simulink model "testmodel_gUSBampCSPbci_TwoClass_gOrthosis"  (R2015a)
settings: Solver=FixedStepDiscrete  StartTime=0.0  StopTime=inf  FixedStep=1/256  RelTol=1e-3
InitFcn:
  | global FeedbackGain;
  | FeedbackGain = 0.1;
  | 
  | if exist('WV') ~= 1
  | global WV
  | WV = zeros(1, 5);
  | end
  | 
  | SelectedChannels = str2num(get_param([gcs,'/Select Channels'],'selectedchannels'));
  | NumberOfChannels = length(SelectedChannels);
  | if (exist('W_CSP') ~= 1)
  |     global W_CSP
  |     if NumberOfChannels == 63
  |         try
  |            SPF = spf;
  |            Filter=load(SPF,'generic_CSP_2Class_63channels.mat');
  |            sf = get(Filter,'spf');
  |            spf_struct = struct(sf);
  |            W_CSP = spf_struct.D.W;
  |         catch
  |             W_CSP = zeros(NumberOfChannels,NumberOfChannels);
  |         end
  |     elseif NumberOfChannels == 27
  |         try
  |             W_CSPt = load('template_W_CSP_TwoClasses_27Ch');
  |             W_CSP = W_CSPt.W_CSP;
  |         catch
  |             W_CSP = zeros(NumberOfChannels,NumberOfChannels);
  |         end
  | elseif NumberOfChannels == 16
  |         try
  |             W_CSPt = load('template_W_CSP_TwoClasses_16Ch');
  |             W_CSP = W_CSPt.W_CSP;
  |         catch
  |             W_CSP = zeros(NumberOfChannels,NumberOfChannels);
  |         end
  |     else
  |         W_CSP = zeros(NumberOfChannels,NumberOfChannels);
  |     end
  | end
StartFcn:
  | SelectedChannels = str2num(get_param([gcs,'/Select Channels'],'selectedchannels'));
  | NumberOfChannels = length(SelectedChannels);
  | 
  | NumCsps = size(W_CSP,1);
  | 
  | if (NumCsps ~= NumberOfChannels)
  | troubles('The number of selected channels does not fit to the number of channels used for setting up the CSPs',['Select the channels in the Select Channels -block to get ',num2str(NumCsps),' channels. If you have changed the electrode configuration please restart Matlab.']);
  | set_param(gcs, 'SimulationCommand', 'stop');
  | end
undefined symbols (not defined in the file or in its folder): Filtera, Filterb
libraries: gRTanalyze x5, gtecHighspeedLib x5, recoveriXExtension_Lib x2, OrthosisLib x1
Description:
  | g.USBamp based CSP MI BCI for two classes
  | 
  | Copyright g.tec medical engineering GmbH
settings Model: ModifiedByFormat=g.tec  CovSFcnEnable=off  Creator=g.tec medical engineering GmbH  LastModifiedBy=g.tec
settings DataIOCC: SignalLoggingSaveFormat=ModelDataLogs
settings OptimizationCC: BlockReduction=off  ExpressionDepthLimit=2147483647  InitFltsAndDblsToZero=on
settings DebuggingCC: SaveWithParameterizedLinksMsg=none  UnderspecifiedInitializationDetection=Classic  MergeDetectMultiDrivingBlocksExec=none  SolverPrmCheckMsg=warning  FcnCallInpInsideContextMsg=UseLocalSettings  StateNameClashWarn=warning
settings GRTTargetCC: CombineOutputUpdateFcns=off  GRTInterface=on

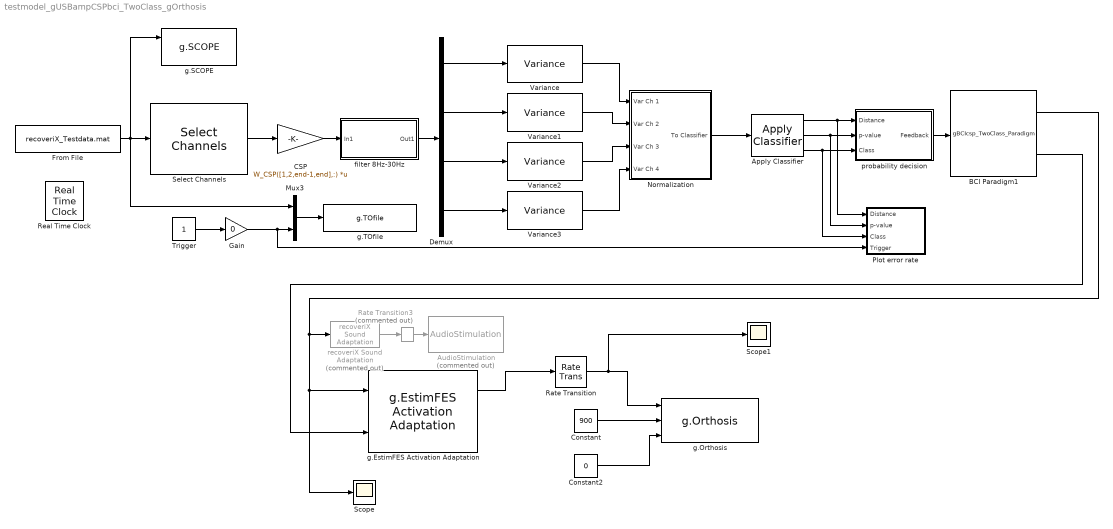
== system testmodel_gUSBampCSPbci_TwoClass_gOrthosis ==
  Apply Classifier : gRTanalyze/Apply Classifier
  AudioStimulation : gtecHighspeedLib/AudioStimulation  Commented=on  audiofiles={'C:\Program Files\gtec\recoveriX g.EstimFES\AudioFiles\Italian\left_resampled.wav' 'C:\Program Files\gtec\recoveriX g.EstimFES\AudioFiles\Italian\right_resampled.wav' 'C:\Program Files\gtec\recoveriX g.EstimFES\AudioFiles\Italian\relax_resampled.wav'}  onsettrigger=0
  BCI Paradigm1 : M-S-Function  FunctionName=gBCIcsp_TwoClass_Paradigm  Parameters=paradigm, runnumber  mask(BCI Paradigm Block){paradigm=feedback, runnumber=1}
      mask TypeOptions paradigm: no feedback | feedback | ball
      mask TypeOptions runnumber: 1 | 2 | 3 | 4
      mask Display:
      | image(imread('feedback_symb.tif'))
      | port_label('output', 1, 'Target');
      | port_label('output', 2, 'Feedback');
      | port_label('input', 1, 'Feedback');
  CSP : Gain  Gain=W_CSP([1,2,end-1,end],:)  Multiplication=Matrix(K*u) (u vector)
  Constant : Constant  Value=900
  Constant2 : Constant  Value=0
  Demux : Demux
  From File : FromFile  FileName=recoveriX_Testdata.mat  SampleTime=1/256
  Gain : Gain  Gain=0
  Mux3 : Mux  Inputs=2
  Normalization : Subsystem
  Plot error rate : Subsystem
  Rate Transition : RateTransition  OutPortSampleTime=128/256
  Rate Transition3 : RateTransition  Commented=on  OutPortSampleTime=1/256
  Real Time Clock : gtecHighspeedLib/Real Time Clock  timeprofile=off
  Scope : Scope
  Scope1 : Scope
  Select Channels : gtecHighspeedLib/Select Channels  selectedchannels="[1   2   3   4   5   6   7   8   9  10  11  12  13  14  15  16]"  totalchannels=17
  Trigger : Constant  SampleTime=1/256
  Variance{,1..3} (4 alike) : gRTanalyze/Variance  WindowLength=384
  filter 8Hz-30Hz : Subsystem  mask{N=5, F_low=8, F_high=30}
      mask prompts: N "Filter order"; F_low "Lower cut-off frequency"; F_high "Upper cut-off frequency"
      mask init:
      | Parent = get_param(gcs, 'Parent');
      | if isempty(Parent)
      | 	Parent = gcs;
      | end
      | 
      | set_param(gcb, 'BackgroundColor', 'darkgreen')
      | set_param(Parent, 'Solver', 'FixedStepDiscrete')
      | pos = get_param(gcb, 'Position');
      | set_param(gcb, 'Position',[pos(1) pos(2) (pos(1)+100) (pos(2)+50)])
      | 
      | if isempty(str2num(get_param(Parent, 'FixedStep')))
      |     % Fixed-step size holds a string.
      |     SamplingTime = get_param(Parent, 'FixedStep');
      |     SampleTime = evalin('base', SamplingTime);
      | else
      |     % Fixed-step size holds a scalar. 
      |     SampleTime = eval(get_param(Parent, 'FixedStep'));
      | end
      | [Filterb,Filtera] = butter(str2num(N),[str2num(F_low),str2num(F_high)].*SampleTime*2,'bandpass');
      | % [b,a] = butter(N,[F_low,F_high].*SampleTime*2);
  g.EstimFES Activation Adaptation : recoveriXExtension_Lib/g.EstimFES Activation Adaptation  stimMode=PRACTICE
  g.Orthosis : OrthosisLib/g.Orthosis  comPort='COM3'
  g.SCOPE : gtecHighspeedLib/g.SCOPE
  g.TOfile : gtecHighspeedLib/g.TOfile  filename=test.mat  varname=y  filesize=100  blocksize=512  enable=off  save_model=off  patient_data=off  id=ID0000  firstname=John  lastname=Doe  dateofbirth=12.01.2001  sex=MALE  hand=RIGHT  diagnosis=Diagnosis  medication=Medication Text  comments=any text ...  run=1  session=1
  probability decision : Subsystem
  recoveriX Sound Adaptation : recoveriXExtension_Lib/recoveriX Sound Adaptation  Commented=on
  wires:
  Demux/1 -> Variance/1
  Demux/3 -> Variance2/1
  Demux/4 -> Variance3/1
  Demux/2 -> Variance1/1
  Variance/1 -> Normalization/1(Var Ch 1)
  Variance2/1 -> Normalization/3(Var Ch 3)
  Variance3/1 -> Normalization/4(Var Ch 4)
  Mux3/1 -> g.TOfile/1
  Normalization/1(To Classifier) -> Apply Classifier/1
  Variance1/1 -> Normalization/2(Var Ch 2)
  From File/1 -> g.SCOPE/1, Select Channels/1, Mux3/1
  Trigger/1 -> Gain/1
  Gain/1 -> Mux3/2, Plot error rate/4(Trigger)
  Apply Classifier/2 -> Plot error rate/2(p-value), probability decision/2(p-value)
  Apply Classifier/3 -> probability decision/3(Class), Plot error rate/3(Class)
  Apply Classifier/1 -> probability decision/1(Distance), Plot error rate/1(Distance)
  probability decision/1(Feedback) -> BCI Paradigm1/1
  CSP/1 -> filter 8Hz-30Hz/1(In1)
  filter 8Hz-30Hz/1(Out1) -> Demux/1
  Select Channels/1 -> CSP/1
  BCI Paradigm1/1 -> recoveriX Sound Adaptation/1, g.EstimFES Activation Adaptation/1, Scope/1
  BCI Paradigm1/2 -> g.EstimFES Activation Adaptation/2
  Constant/1 -> g.Orthosis/2
  recoveriX Sound Adaptation/1 -> Rate Transition3/1
  Rate Transition3/1 -> AudioStimulation/1
  Constant2/1 -> g.Orthosis/3
  g.EstimFES Activation Adaptation/1 -> Rate Transition/1
  Rate Transition/1 -> Scope1/1, g.Orthosis/1

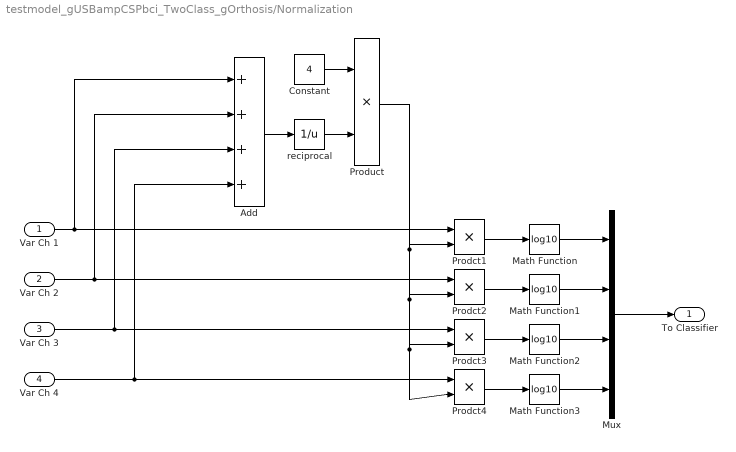
== system testmodel_gUSBampCSPbci_TwoClass_gOrthosis/Normalization ==
  Var Ch 1 : Inport
  Var Ch 2 : Inport  Port=2
  Var Ch 3 : Inport  Port=3
  Var Ch 4 : Inport  Port=4
  Add : Sum  Inputs=++++
  Constant : Constant  Value=4
  Math Function{,1..3} (4 alike) : Math  Operator=log10  SaturateOnIntegerOverflow=on
  Mux : Mux
  Prodct{1..4} (4 alike) : Product  RndMeth=Zero
  Product : Product  RndMeth=Zero
  reciprocal : Math  Operator=reciprocal  SaturateOnIntegerOverflow=on
  To Classifier : Outport
  wires:
  Var Ch 1/1 -> Add/1, Prodct1/1
  Var Ch 3/1 -> Add/3, Prodct3/1
  Var Ch 4/1 -> Add/4, Prodct4/1
  Constant/1 -> Product/1
  reciprocal/1 -> Product/2
  Var Ch 2/1 -> Add/2, Prodct2/1
  Add/1 -> reciprocal/1
  Prodct1/1 -> Math Function/1
  Prodct2/1 -> Math Function1/1
  Prodct3/1 -> Math Function2/1
  Prodct4/1 -> Math Function3/1
  Product/1 -> Prodct4/2, Prodct3/2, Prodct2/2, Prodct1/2
  Math Function/1 -> Mux/1
  Math Function1/1 -> Mux/2
  Math Function2/1 -> Mux/3
  Math Function3/1 -> Mux/4
  Mux/1 -> To Classifier/1

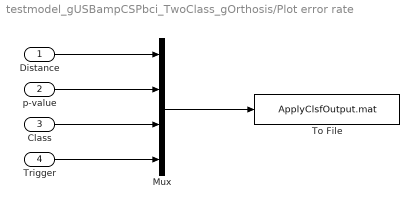
== system testmodel_gUSBampCSPbci_TwoClass_gOrthosis/Plot error rate ==
  Distance : Inport
  p-value : Inport  Port=2
  Class : Inport  Port=3
  Trigger : Inport  Port=4
  Mux : Mux
  To File : ToFile  Filename=ApplyClsfOutput.mat  MatrixName=y
  wires:
  Distance/1 -> Mux/1
  p-value/1 -> Mux/2
  Class/1 -> Mux/3
  Trigger/1 -> Mux/4
  Mux/1 -> To File/1

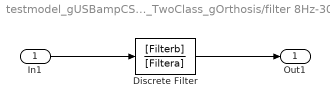
== system testmodel_gUSBampCSPbci_TwoClass_gOrthosis/filter 8Hz-30Hz ==
  In1 : Inport
  Discrete Filter : DiscreteFilter  Numerator=[Filterb]  Denominator=[Filtera]
  Out1 : Outport
  wires:
  Discrete Filter/1 -> Out1/1
  In1/1 -> Discrete Filter/1

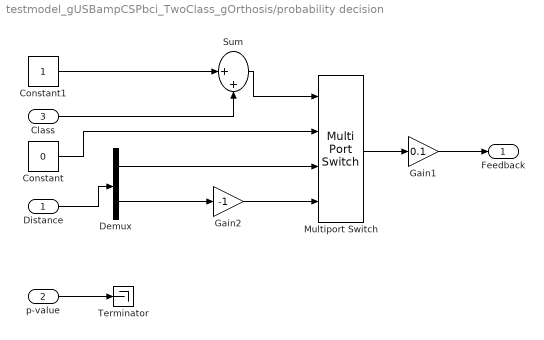
== system testmodel_gUSBampCSPbci_TwoClass_gOrthosis/probability decision ==
  Distance : Inport
  p-value : Inport  Port=2
  Class : Inport  Port=3
  Constant : Constant  Value=0
  Constant1 : Constant
  Demux : Demux  Outputs=2
  Gain1 : Gain  Gain=0.1
  Gain2 : Gain  Gain=-1
  Multiport Switch : MultiPortSwitch
  Sum : Sum  Inputs=|++
  Terminator : Terminator
  Feedback : Outport
  wires:
  Gain1/1 -> Feedback/1
  Distance/1 -> Demux/1
  Demux/2 -> Gain2/1
  Multiport Switch/1 -> Gain1/1
  Sum/1 -> Multiport Switch/1
  Gain2/1 -> Multiport Switch/4
  Demux/1 -> Multiport Switch/3
  Constant/1 -> Multiport Switch/2
  p-value/1 -> Terminator/1
  Class/1 -> Sum/2
  Constant1/1 -> Sum/1
